simulink model "three_body_P_matlab_function"  (R2023b)
settings: Solver=ode4  StartTime=0.0  StopTime=20  FixedStep=0.001  RelTol=1e-3
values from neighbouring files (symbols this model uses):
  dot_X0 = trajectory(1, 4:5)    [init.m]
  trajectory = readmatrix("trajectory.csv")    [init.m]    (also in ploter.m)
  X0 = trajectory(1, 1:2)    [init.m]
libraries: slpidlib x1
settings Model: Creator=Ali  LastModifiedBy=Ali

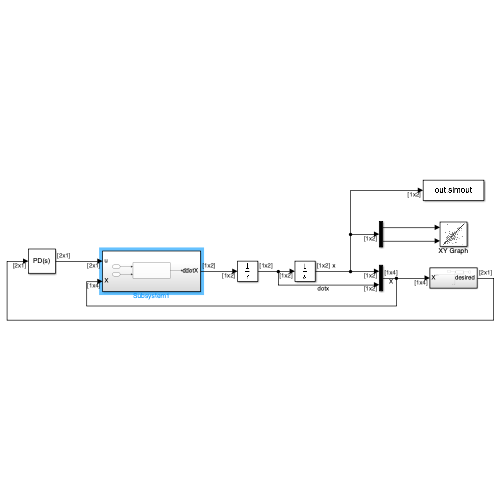
[thumbnail: Simulink's stored preview of the top-level diagram]
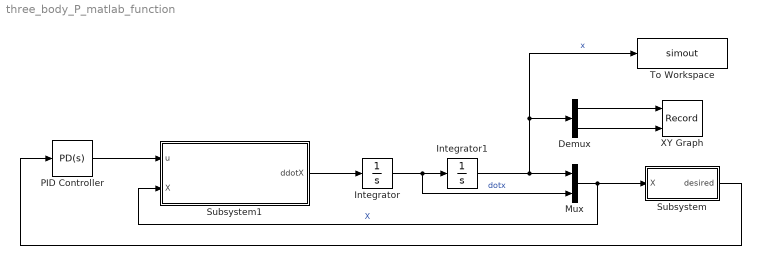
== system three_body_P_matlab_function ==
  Demux : Demux  Outputs=2
  Integrator : Integrator  InitialCondition=dot_X0
  Integrator1 : Integrator  InitialCondition=X0
  Mux : Mux  Inputs=2
  PID Controller : slpidlib/PID Controller  Controller=PD  Form=Parallel  TimeDomain=Continuous-time  UseExternalTs=off  SampleTime=-1  IntegratorMethod=Forward Euler  FilterMethod=Forward Euler  ControllerParametersSource=internal  P=10  I=0  UseKiTs=off  D=10  N=100  UseFilter=on  TunerSelectOption=Transfer Function Based (PID Tuner App)  InitialConditionSource=internal  InitialConditionForIntegrator=0  InitialConditionForFilter=0  DifferentiatorICPrevScaledInput=0  ExternalReset=none  TrackingMode=off  Kt=1  LimitOutput=off  SatLimitsSource=internal  UpperSaturationLimit=inf  LowerSaturationLimit=-inf  LinearizeAsGain=on  AntiWindupMode=none  Kb=1  LimitIntegrator=off  UpperIntegratorSaturationLimit=inf  LowerIntegratorSaturationLimit=-inf  POutMin=[]  POutMax=[]  IOutMin=[]  IOutMax=[]  DOutMin=[]  DOutMax=[]  NOutMin=[]  NOutMax=[]  SumOutMin=[]  SumOutMax=[]  SaturationOutMin=[]  SaturationOutMax=[]  PParamMin=[]  PParamMax=[]  IParamMin=[]  IParamMax=[]  DParamMin=[]  DParamMax=[]  NParamMin=[]  NParamMax=[]  KbParamMin=[]  KbParamMax=[]  KtParamMin=[]  KtParamMax=[]  KbOutMin=[]  KbOutMax=[]  KtOutMin=[]  KtOutMax=[]  IntegratorOutMin=[]  IntegratorOutMax=[]  FilterOutMin=[]  FilterOutMax=[]  SumI1OutMin=[]  SumI1OutMax=[]  SumI2OutMin=[]  SumI2OutMax=[]  SumI3OutMin=[]  SumI3OutMax=[]  SumI4OutMin=[]  SumI4OutMax=[]  SumDOutMin=[]  SumDOutMax=[]  DifferentiatorOutMin=[]  DifferentiatorOutMax=[]  FilterDiffOutCoefMin=[]  FilterDiffOutCoefMax=[]  ReciprocalOutMin=[]  ReciprocalOutMax=[]  SumDenOutMin=[]  SumDenOutMax=[]  SumNumOutMin=[]  SumNumOutMax=[]  DivideOutMin=[]  DivideOutMax=[]  UdiffTsProdOutMin=[]  UdiffTsProdOutMax=[]  NTsProdOutMin=[]  NTsProdOutMax=[]  UintegralTsProdOutMin=[]  UintegralTsProdOutMax=[]  UngainTsProdOutMin=[]  UngainTsProdOutMax=[]  ClampingZeroOutDataTypeStr=Inherit: Inherit via back propagation  ClampingZeroOutMin=[]  ClampingZeroOutMax=[]  FilterDenConstantOutDataTypeStr=Inherit: Inherit via back propagation  FilterDenConstantOutMin=[]  FilterDenConstantOutMax=[]  PCopyOutDataTypeStr=Inherit: Inherit via back propagation  PCopyOutMin=[]  PCopyOutMax=[]  NCopyOutDataTypeStr=Inherit: Inherit via back propagation  NCopyOutMin=[]  NCopyOutMax=[]  IntegratorContinuousStateAttributes=''  IntegratorStateMustResolveToSignalObject=off  IntegratorRTWStateStorageClass=Auto  FilterContinuousStateAttributes=''  FilterStateMustResolveToSignalObject=off  FilterRTWStateStorageClass=Auto  ParallelPVariant=InternalParameters  IdealPVariant=Disabled  IVariant=Disabled  DVariant=InternalParameters  IntegratorVariant=Disabled  SatVariant=Disabled  AWVariant=Disabled  PCopyVariant=Disabled  TRVariant=Disabled  FdbkBlocksVariant=Forward  IdealPFdbkVariant=Disabled  SatFdbkVariant=Disabled  DerivativeFilterVariant=ContFilter  NVariant=InternalParameters  NCopyVariant=Disabled  FilterICVariant=InternalICsFilter  IntegratorICVariant=Disabled  ExternalResetVariant=Disabled  TRSumVariant=Passthrough  SumFdbkVariant=Disabled  SumVariant=Sum_PD  TsampFilterVariant=InternalTs  TsampNgainVariant=Passthrough  TsampIntegralVariant=Disabled_SignalSpec  ExternalSaturationOutDataTypeStr=Inherit: Same as second input
  Subsystem : Subsystem
  Subsystem1 : Subsystem
  To Workspace : ToWorkspace  VariableName=simout  SampleTime=-1
      settings: Save2DSignal=2-D array (concatenate along first dimension)
  XY Graph : Record  FileSettingsInternal="{\"entries\":[{\"content\":{\"excelSettings\":{\"content\":{},\"type\":\"Streamout.ExcelSettings\"}},\"type\":\"Streamout.FileSettingStorage\",\"uuid\":\"\"}],\"packageUris\":[\"http:\\/\\/schema.mathworks.com\\/mf0\\/streamout_blocks\\/R2020a\"],\"version\":\"1.0\"}"  Layout=[1 1]  SignalsInternal="{\"entries\":[{\"content\":{\"signals\":[{\"content\":{\"blockPath\":[],\"dimensions\":[1,1],\"domain\":\"\",\"lineColor\":\"#a2142f\",\"plots\":[1],\"port\":1,\"sid\":[\"\"],\"signalID\":5052,\"signalName\":\"Demux:1\"},\"type\":\"RecordBlkView.Signal\",\"uuid\":\"\"},{\"content\":{\"blockPath\":[],\"dimensions\":[1,1],\"domain\":\"\",\"lineColor\":\"#139fff\",\"plots\":[1],\"port\":2,\"sid\":[\"\"],\"signalID\":5056,\"signalName\":\"Demux:2\"},\"type\":\"RecordBlkView.Signal\",\"uuid\":\"\"}]},\"type\":\"RecordBlkView.InputSignals\",\"uuid\":\"\"}],\"packageUris\":[\"http:\\/\\/schema.mathworks.com\\/mf0\\/streamout_blocks\\/R2020a\"],\"version\":\"1.0\"}"  VisualizationBindings="{\"xyplotplugin\":{\"info\":[{\"series\":[{\"bindingParametersList\":[{\"parameter\":\"X-Axis\",\"signalID\":5052,\"signalName\":\"Demux:1\"},{\"parameter\":\"Y-Axis\",\"signalID\":5056,\"signalName\":\"Demux:2\"}],\"seriesID\":9120}],\"subplotID\":1}]}}"  CompatibilityTag=XY
  wires:
  Integrator1/1 -> To Workspace/1, Demux/1, Mux/1  "x"
  Demux/1 -> XY Graph/1
  Demux/2 -> XY Graph/2
  Mux/1 -> Subsystem1/2(X), Subsystem/1(X)  "X"
  Integrator/1 -> Mux/2, Integrator1/1  "dotx"
  Subsystem/1(desired) -> PID Controller/1
  PID Controller/1 -> Subsystem1/1(u)
  Subsystem1/1(ddotX) -> Integrator/1

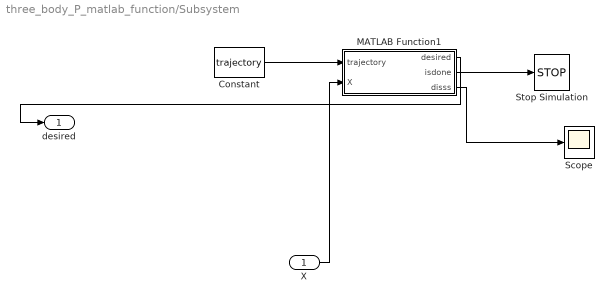
== system three_body_P_matlab_function/Subsystem ==
  X : Inport
  Constant : Constant  Value=trajectory
  MATLAB Function1 : MATLAB Function  TreatAsAtomicUnit=on
  Scope : Scope
  Stop Simulation : Stop
  desired : Outport
  wires:
  MATLAB Function1/1(desired) -> desired/1
  Constant/1 -> MATLAB Function1/1(trajectory)
  X/1 -> MATLAB Function1/2(X)
  MATLAB Function1/3(disss) -> Scope/1
  MATLAB Function1/2(isdone) -> Stop Simulation/1

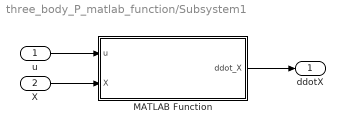
== system three_body_P_matlab_function/Subsystem1 ==
  u : Inport
  X : Inport  Port=2
  MATLAB Function : MATLAB Function  TreatAsAtomicUnit=on
  ddotX : Outport
  wires:
  X/1 -> MATLAB Function/2(X)
  u/1 -> MATLAB Function/1(u)
  MATLAB Function/1(ddot_X) -> ddotX/1

== matlab function three_body_P_matlab_function/Subsystem/MATLAB Function1 ==
  settings: updateMethod=DISCRETE
  data: trajectory input; desired output size=[2, 1]; X input; isdone output; disss output
function [desired, isdone, disss] = fcn(trajectory, X)

persistent point_index
if isempty(point_index)
    point_index = 0;
end

trajectory = trajectory(:, 1:2)';
xy = X(1:2);
distance = ((trajectory - xy).^2);
dist = sum(distance);
dist = dist';
index = find(dist==min(dist));
index = index(1);
if index <= point_index && index < length(trajectory)
    index = point_index + 1;
end
point_index = index;
if index > length(trajectory)
    index = length(trajectory);
end
answer = trajectory(:, index);
t = reshape(xy, [2, 1]);
desired = reshape(answer, [2, 1]) - t;
desired = desired * 100;

isdone = false;
final_point = trajectory(:, end);
disss = sqrt(sum((xy - final_point).^2));
if disss <= 0.005
    isdone = true;
end

== matlab function three_body_P_matlab_function/Subsystem1/MATLAB Function ==
  data: u input; ddot_X output; X input
function ddot_X = fcn(u, X)

mu = 0.012277471;

a_x = u(1);
a_y = u(2);

% Positions
x = X(1);
y = X(2);
z = 0;
% Velocities
xdot = X(3);
ydot = X(4);

% distances from particle to primaries
r1 = sqrt((x+mu)^2 + y^2 + z^2); 
r2 = sqrt((x-1+mu)^2 + y^2 + z^2); 

% Accelerations 
xddot = 2*ydot + x -(1-mu)*((x+mu)/(r1^3)) - mu*(x-1+mu)/(r2^3) + a_x;
yddot = -2*xdot + y - (1-mu)*(y/(r1^3)) - mu*(y)/(r2^3) + a_y;

ddot_X = [xddot; yddot]';
